simulink model "item3ModeloNLinPS"  (R2017a)
settings: Solver=VariableStepAuto  StartTime=0.0  StopTime=100  RelTol=1e-3
values from neighbouring files (symbols this model uses):
  C_d = minreal(c2d(C, Ts, 'matched'))    [Item3PSF.m]    (also in item3_PSF_comK.m = c2d(C, Ts, 'matched'); psfRapido.m)
  F_d = minreal(c2d(F, Ts, 'matched'))    [Item3PSF.m]    (also in item3_PSF_comK.m = c2d(F, Ts, 'matched'); psfRapido.m)
  Fr = minreal((NumFr/DenFr),1e-2)    [Item3PSF.m]    (also in item3_PSF_comK.m = ((alpha*(z^2) + beta*z + gamma)*(K)*(z^2 - 1.628*z + 0.7312); psfRapido.m = minreal(NumFr/DenFr); robustezPSF.m = minreal(NumFr/DenFr))
  Gu_d = minreal(c2d(Gu, Ts, 'zoh'))    [Item3PSF.m]    (also in item3_PSF_comK.m = c2d(Gu, Ts, 'zoh'); psfRapido.m)
  Ts = t_5/20    (= 0.075)    [Item3PSF.m]    (also in item3_PSF_comK.m; psfRapido.m; robustezPSF.m)
libraries: simulink x4
settings Model: Creator=julia  LastModifiedBy=julia

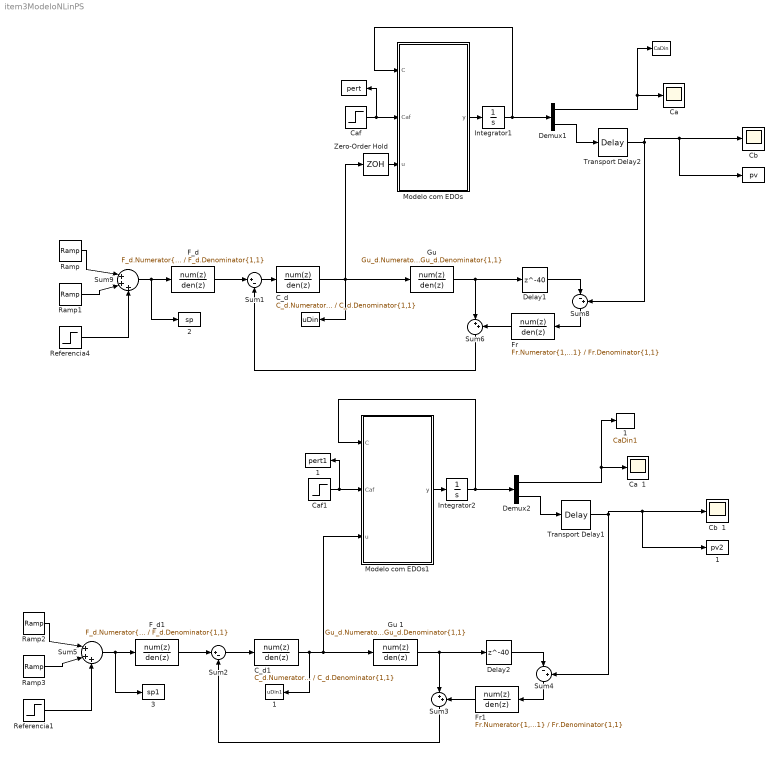
== system item3ModeloNLinPS ==
  "   " : ToWorkspace  VariableName=pv  SaveFormat=Timeseries  SampleTime=-1
  "          " : ToWorkspace  VariableName=pert  SaveFormat=Timeseries  SampleTime=-1
  "                 " : ToWorkspace  VariableName=uDin  SaveFormat=Timeseries  SampleTime=-1
  "                   " : ToWorkspace  VariableName=CaDin  SaveFormat=Timeseries  SampleTime=-1
  "                   1" : ToWorkspace  VariableName=CaDin1  SaveFormat=Timeseries  SampleTime=-1
  "                 1" : ToWorkspace  VariableName=uDin1  SaveFormat=Timeseries  SampleTime=-1
  "          1" : ToWorkspace  VariableName=pert1  SaveFormat=Timeseries  SampleTime=-1
  "   1" : ToWorkspace  VariableName=pv2  SaveFormat=Timeseries  SampleTime=-1
  "   2" : ToWorkspace  VariableName=sp  SaveFormat=Timeseries  SampleTime=-1
  "   3" : ToWorkspace  VariableName=sp1  SaveFormat=Timeseries  SampleTime=-1
  C_d : DiscreteTransferFcn  Numerator=C_d.Numerator{1,1}  Denominator=C_d.Denominator{1,1}  SampleTime=Ts
  C_d1 : DiscreteTransferFcn  Numerator=C_d.Numerator{1,1}  Denominator=C_d.Denominator{1,1}  SampleTime=Ts
  "Ca  " : Scope
  Ca  1 : Scope
  Caf : Step  Time=60  Before=5.1  After=5.15  SampleTime=0
  Caf1 : Step  Time=60  Before=5.1  After=5.15  SampleTime=0
  "Cb  " : Scope
  Cb  1 : Scope
  Delay1 : Delay  DelayLength=40  InitialCondition=0
  Delay2 : Delay  DelayLength=40  InitialCondition=0
  Demux1 : Demux  Outputs=2
  Demux2 : Demux  Outputs=2
  F_d : DiscreteTransferFcn  Numerator=F_d.Numerator{1,1}  Denominator=F_d.Denominator{1,1}  SampleTime=Ts
  F_d1 : DiscreteTransferFcn  Numerator=F_d.Numerator{1,1}  Denominator=F_d.Denominator{1,1}  SampleTime=Ts
  Fr : DiscreteTransferFcn  Numerator=Fr.Numerator{1,1}  Denominator=Fr.Denominator{1,1}  SampleTime=Ts
  Fr1 : DiscreteTransferFcn  Numerator=Fr.Numerator{1,1}  Denominator=Fr.Denominator{1,1}  SampleTime=Ts
  "Gu " : DiscreteTransferFcn  Numerator=Gu_d.Numerator{1,1}  Denominator=Gu_d.Denominator{1,1}  SampleTime=Ts
  Gu 1 : DiscreteTransferFcn  Numerator=Gu_d.Numerator{1,1}  Denominator=Gu_d.Denominator{1,1}  SampleTime=Ts
  Integrator1 : Integrator  InitialCondition=[0;0]
  Integrator2 : Integrator  InitialCondition=[0;0]
  Modelo com EDOs : MATLAB Function  TreatAsAtomicUnit=on
  Modelo com EDOs1 : MATLAB Function  TreatAsAtomicUnit=on
  Ramp : simulink/Sources/Ramp  slope=2.345/10  start=0  X0=0
  Ramp1 : simulink/Sources/Ramp  slope=-2.345/10  start=10  X0=0
  Ramp2 : simulink/Sources/Ramp  slope=2.345/10  start=0  X0=0
  Ramp3 : simulink/Sources/Ramp  slope=-2.345/10  start=10  X0=0
  Referencia1 : Step  Time=30  After=0.35  SampleTime=0
  Referencia4 : Step  Time=30  After=0.1  SampleTime=0
  Sum1 : Sum  Inputs=|+-
  Sum2 : Sum  Inputs=|+-
  Sum3 : Sum  Inputs=|++
  Sum4 : Sum  Inputs=|-+
  Sum5 : Sum  Inputs=|+++
  Sum6 : Sum  Inputs=|++
  Sum8 : Sum  Inputs=|-+
  Sum9 : Sum  Inputs=|+++
  Transport Delay1 : TransportDelay  DelayTime=3
  Transport Delay2 : TransportDelay  DelayTime=3
  Zero-Order Hold : ZeroOrderHold  SampleTime=Ts
  wires:
  Modelo com EDOs/1(y) -> Integrator1/1
  Integrator1/1 -> Modelo com EDOs/1(C), Demux1/1
  Demux1/1 -> "                   "/1, "Ca  "/1
  Caf/1 -> "          "/1, Modelo com EDOs/2(Caf)
  Referencia4/1 -> Sum9/3
  Ramp1/1 -> Sum9/2
  Ramp/1 -> Sum9/1
  Demux1/2 -> Transport Delay2/1
  F_d/1 -> Sum1/1
  Sum8/1 -> Fr/1
  Sum6/1 -> Sum1/2
  C_d/1 -> Zero-Order Hold/1, "                 "/1, "Gu "/1
  Sum9/1 -> "   2"/1, F_d/1
  Fr/1 -> Sum6/2
  "Gu "/1 -> Sum6/1, Delay1/1
  Delay1/1 -> Sum8/1
  Sum1/1 -> C_d/1
  Transport Delay2/1 -> "   "/1, "Cb  "/1, Sum8/2
  Transport Delay1/1 -> Sum4/2, Cb  1/1, "   1"/1
  Sum2/1 -> C_d1/1
  Delay2/1 -> Sum4/1
  Gu 1/1 -> Delay2/1, Sum3/1
  Fr1/1 -> Sum3/2
  Sum5/1 -> F_d1/1, "   3"/1
  C_d1/1 -> Gu 1/1, Modelo com EDOs1/3(u), "                 1"/1
  Sum3/1 -> Sum2/2
  Sum4/1 -> Fr1/1
  F_d1/1 -> Sum2/1
  Demux2/2 -> Transport Delay1/1
  Ramp2/1 -> Sum5/1
  Ramp3/1 -> Sum5/2
  Referencia1/1 -> Sum5/3
  Caf1/1 -> Modelo com EDOs1/2(Caf), "          1"/1
  Demux2/1 -> Ca  1/1, "                   1"/1
  Integrator2/1 -> Demux2/1, Modelo com EDOs1/1(C)
  Modelo com EDOs1/1(y) -> Integrator2/1
  Zero-Order Hold/1 -> Modelo com EDOs/3(u)

== matlab function item3ModeloNLinPS/Modelo com EDOs ==
  data: y output; C input; Caf input; u input
%EDOs das concentracoes dos produtos A e B
function y = fcn(C, Caf, u)

%constantes
k1 = 6.01; %L/min
k2 = 0.8433; %L/min
k3 = 0.1123; %mol/Lmin

%variaveis das concentracoes dos produtos A e B
Ca = C(1);
Cb = C(2);

%EDOs
Ca_d = -k1*Ca - k3*(Ca^2) + (Caf - Ca)*u;
Cb_d =  k1*Ca - k2*Cb - Cb*u;
 
%conjunto das EDOs
y = [Ca_d;Cb_d];

== matlab function item3ModeloNLinPS/Modelo com EDOs1 ==
  data: y output; C input; Caf input; u input
%EDOs das concentracoes dos produtos A e B
function y = fcn(C, Caf, u)

%constantes
k1 = 6.01; %L/min
k2 = 0.8433; %L/min
k3 = 0.1123; %mol/Lmin

%variaveis das concentracoes dos produtos A e B
Ca = C(1);
Cb = C(2);

%EDOs
Ca_d = -k1*Ca - k3*(Ca^2) + (Caf - Ca)*u;
Cb_d =  k1*Ca - k2*Cb - Cb*u;
 
%conjunto das EDOs
y = [Ca_d;Cb_d];
